simulink model "mbed_stm32stampf446_blinky"  (R2015a)
settings: Solver=FixedStepDiscrete  SolverMode=SingleTasking  StartTime=0.0  StopTime=10.0  FixedStep=1e-3  RelTol=1e-3
libraries: mbed_lib x2
settings Model: CovSFcnEnable=off  Creator=oh  LastModifiedBy=oh
settings OptimizationCC: OptimizeModelRefInitCode=on  LifeSpan=1
settings DebuggingCC: SolverPrmCheckMsg=warning
settings HardwareCC: ProdLargestAtomicInteger=Long  ProdLargestAtomicFloat=Double  ProdEndianess=LittleEndian  ProdHWDeviceType=ARM Compatible->ARM Cortex
settings RTWCC: SystemTargetFile=mbed.tlc  TemplateMakefile=mbed.tmf  Description=Mbed Target (Embedded Target)  TargetLang=C++
settings CodeAppCC: IgnoreCustomStorageClasses=off
settings STFCustomTargetCC: CombineOutputUpdateFcns=on  SupportContinuousTime=off  SupportVariableSizeSignals=off  SystemTargetFile=mbed.tlc
settings ERTTargetCC: SupportContinuousTime=off  SupportVariableSizeSignals=off  ERTCustomFileTemplate=mbed_file_process.tlc

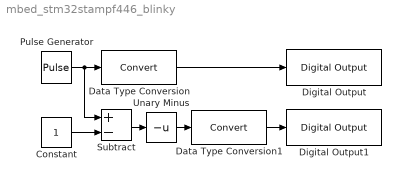
== system mbed_stm32stampf446_blinky ==
  Constant : Constant
  Data Type Conversion : DataTypeConversion
  Data Type Conversion1 : DataTypeConversion
  Digital Output : mbed_lib/GPIO/Digital Output  SParameter2=C  SParameter1=10  SParameter3=PullDefault  SampleTime=-1
  Digital Output1 : mbed_lib/GPIO/Digital Output  SParameter2=C  SParameter1=11  SParameter3=PullDefault  SampleTime=-1
  Pulse Generator : DiscretePulseGenerator  PulseType=Time based  Period=0.5  PulseWidth=50
  Subtract : Sum  Inputs=+-
  Unary Minus : UnaryMinus
  wires:
  Pulse Generator/1 -> Subtract/1, Data Type Conversion/1
  Data Type Conversion/1 -> Digital Output/1
  Constant/1 -> Subtract/2
  Subtract/1 -> Unary Minus/1
  Unary Minus/1 -> Data Type Conversion1/1
  Data Type Conversion1/1 -> Digital Output1/1
